simulink model "final"  (R2022a)
settings: Solver=FixedStepAuto  StartTime=0.0  StopTime=5.0  FixedStep=0.001  RelTol=1e-3
libraries: instrumentseriallib x3, slpidlib x2
settings Model: Creator=13025  LastModifiedBy=13025
settings OptimizationCC: DenormalBehavior=FlushToZero
settings DebuggingCC: ReadBeforeWriteMsg=DisableAll  WriteAfterWriteMsg=DisableAll  WriteAfterReadMsg=DisableAll

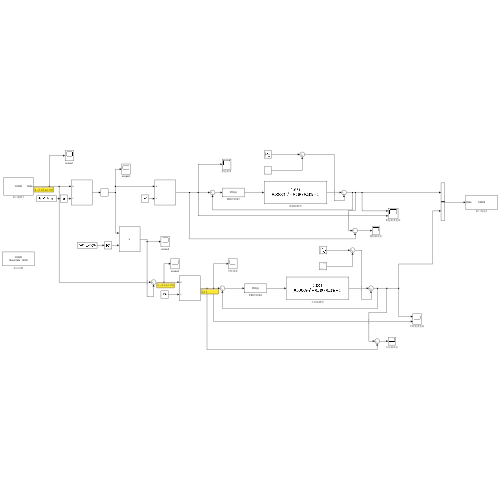
[thumbnail: Simulink's stored preview of the top-level diagram]
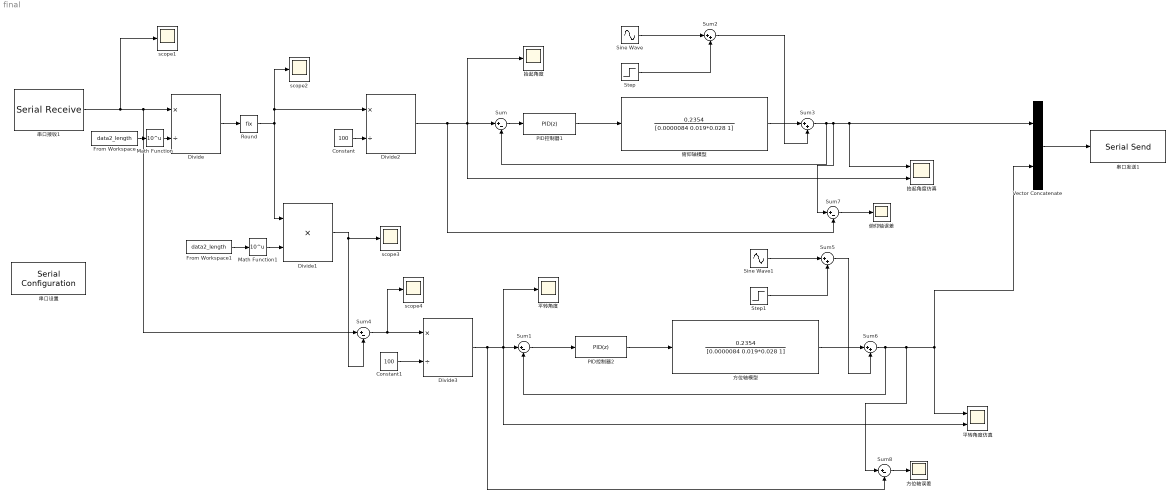
== system final ==
  Constant : Constant  Value=100
  Constant1 : Constant  Value=100
  Divide : Product  Inputs=*/  OutDataTypeStr=single  RndMeth=Round  LockScale=on
  Divide1 : Product  Inputs=**  OutDataTypeStr=single  RndMeth=Nearest  LockScale=on
  Divide2 : Product  Inputs=*/  OutDataTypeStr=double  RndMeth=Simplest
  Divide3 : Product  Inputs=*/  OutDataTypeStr=double
  From Workspace : FromWorkspace  VariableName=data2_length  OutDataTypeStr=double  SampleTime=5  OutputAfterFinalValue=Holding final value
  From Workspace1 : FromWorkspace  VariableName=data2_length  OutDataTypeStr=double  SampleTime=5  OutputAfterFinalValue=Holding final value
  Math Function : Math  Operator=10^u
  Math Function1 : Math  Operator=10^u
  PID控制器1 : slpidlib/PID Controller  Controller=PID  Form=Parallel  TimeDomain=Discrete-time  UseExternalTs=off  SampleTime=-1  IntegratorMethod=Forward Euler  FilterMethod=Forward Euler  ControllerParametersSource=internal  P=1  I=127  UseKiTs=off  D=0  N=100  UseFilter=on  TunerSelectOption=Transfer Function Based (PID Tuner App)  InitialConditionSource=internal  InitialConditionForIntegrator=0  InitialConditionForFilter=0  DifferentiatorICPrevScaledInput=0  ExternalReset=none  TrackingMode=off  Kt=1  LimitOutput=off  SatLimitsSource=internal  UpperSaturationLimit=inf  LowerSaturationLimit=-inf  LinearizeAsGain=on  AntiWindupMode=none  Kb=1  POutMin=[]  POutMax=[]  IOutMin=[]  IOutMax=[]  DOutMin=[]  DOutMax=[]  NOutMin=[]  NOutMax=[]  SumOutMin=[]  SumOutMax=[]  SaturationOutMin=[]  SaturationOutMax=[]  PParamMin=[]  PParamMax=[]  IParamMin=[]  IParamMax=[]  DParamMin=[]  DParamMax=[]  NParamMin=[]  NParamMax=[]  KbParamMin=[]  KbParamMax=[]  KtParamMin=[]  KtParamMax=[]  KbOutMin=[]  KbOutMax=[]  KtOutMin=[]  KtOutMax=[]  IntegratorOutMin=[]  IntegratorOutMax=[]  FilterOutMin=[]  FilterOutMax=[]  SumI1OutMin=[]  SumI1OutMax=[]  SumI2OutMin=[]  SumI2OutMax=[]  SumI3OutMin=[]  SumI3OutMax=[]  SumI4OutMin=[]  SumI4OutMax=[]  SumDOutMin=[]  SumDOutMax=[]  DifferentiatorOutMin=[]  DifferentiatorOutMax=[]  FilterDiffOutCoefMin=[]  FilterDiffOutCoefMax=[]  ReciprocalOutMin=[]  ReciprocalOutMax=[]  SumDenOutMin=[]  SumDenOutMax=[]  SumNumOutMin=[]  SumNumOutMax=[]  DivideOutMin=[]  DivideOutMax=[]  UdiffTsProdOutMin=[]  UdiffTsProdOutMax=[]  NTsProdOutMin=[]  NTsProdOutMax=[]  UintegralTsProdOutMin=[]  UintegralTsProdOutMax=[]  UngainTsProdOutMin=[]  UngainTsProdOutMax=[]  ClampingZeroOutDataTypeStr=Inherit: Inherit via back propagation  ClampingZeroOutMin=[]  ClampingZeroOutMax=[]  FilterDenConstantOutDataTypeStr=Inherit: Inherit via back propagation  FilterDenConstantOutMin=[]  FilterDenConstantOutMax=[]  PCopyOutDataTypeStr=Inherit: Inherit via back propagation  PCopyOutMin=[]  PCopyOutMax=[]  NCopyOutDataTypeStr=Inherit: Inherit via back propagation  NCopyOutMin=[]  NCopyOutMax=[]  IntegratorContinuousStateAttributes=''  IntegratorStateMustResolveToSignalObject=off  IntegratorRTWStateStorageClass=Auto  FilterContinuousStateAttributes=''  FilterStateMustResolveToSignalObject=off  FilterRTWStateStorageClass=Auto  ParallelPVariant=InternalParameters  IdealPVariant=Disabled  IVariant=InternalParameters  DVariant=InternalParameters  IntegratorVariant=Discrete  SatVariant=Disabled  AWVariant=Passthrough  PCopyVariant=Disabled  TRVariant=Disabled  FdbkBlocksVariant=Forward  IdealPFdbkVariant=Disabled  SatFdbkVariant=Disabled  DerivativeFilterVariant=ForwardEulerFilter  NVariant=InternalParameters  NCopyVariant=Disabled  FilterICVariant=InternalICsFilter  IntegratorICVariant=InternalICs  ExternalResetVariant=Disabled  TRSumVariant=Passthrough  SumFdbkVariant=Disabled  SumVariant=Sum_PID  TsampFilterVariant=InternalTs  TsampNgainVariant=Passthrough  TsampIntegralVariant=Passthrough  ExternalSaturationOutDataTypeStr=Inherit: Same as second input  aMode=0
  PID控制器2 : slpidlib/PID Controller  Controller=PID  Form=Parallel  TimeDomain=Discrete-time  UseExternalTs=off  SampleTime=-1  IntegratorMethod=Forward Euler  FilterMethod=Forward Euler  ControllerParametersSource=internal  P=1  I=127  UseKiTs=off  D=0  N=100  UseFilter=on  TunerSelectOption=Transfer Function Based (PID Tuner App)  InitialConditionSource=internal  InitialConditionForIntegrator=0  InitialConditionForFilter=0  DifferentiatorICPrevScaledInput=0  ExternalReset=none  TrackingMode=off  Kt=1  LimitOutput=off  SatLimitsSource=internal  UpperSaturationLimit=inf  LowerSaturationLimit=-inf  LinearizeAsGain=on  AntiWindupMode=none  Kb=1  POutMin=[]  POutMax=[]  IOutMin=[]  IOutMax=[]  DOutMin=[]  DOutMax=[]  NOutMin=[]  NOutMax=[]  SumOutMin=[]  SumOutMax=[]  SaturationOutMin=[]  SaturationOutMax=[]  PParamMin=[]  PParamMax=[]  IParamMin=[]  IParamMax=[]  DParamMin=[]  DParamMax=[]  NParamMin=[]  NParamMax=[]  KbParamMin=[]  KbParamMax=[]  KtParamMin=[]  KtParamMax=[]  KbOutMin=[]  KbOutMax=[]  KtOutMin=[]  KtOutMax=[]  IntegratorOutMin=[]  IntegratorOutMax=[]  FilterOutMin=[]  FilterOutMax=[]  SumI1OutMin=[]  SumI1OutMax=[]  SumI2OutMin=[]  SumI2OutMax=[]  SumI3OutMin=[]  SumI3OutMax=[]  SumI4OutMin=[]  SumI4OutMax=[]  SumDOutMin=[]  SumDOutMax=[]  DifferentiatorOutMin=[]  DifferentiatorOutMax=[]  FilterDiffOutCoefMin=[]  FilterDiffOutCoefMax=[]  ReciprocalOutMin=[]  ReciprocalOutMax=[]  SumDenOutMin=[]  SumDenOutMax=[]  SumNumOutMin=[]  SumNumOutMax=[]  DivideOutMin=[]  DivideOutMax=[]  UdiffTsProdOutMin=[]  UdiffTsProdOutMax=[]  NTsProdOutMin=[]  NTsProdOutMax=[]  UintegralTsProdOutMin=[]  UintegralTsProdOutMax=[]  UngainTsProdOutMin=[]  UngainTsProdOutMax=[]  ClampingZeroOutDataTypeStr=Inherit: Inherit via back propagation  ClampingZeroOutMin=[]  ClampingZeroOutMax=[]  FilterDenConstantOutDataTypeStr=Inherit: Inherit via back propagation  FilterDenConstantOutMin=[]  FilterDenConstantOutMax=[]  PCopyOutDataTypeStr=Inherit: Inherit via back propagation  PCopyOutMin=[]  PCopyOutMax=[]  NCopyOutDataTypeStr=Inherit: Inherit via back propagation  NCopyOutMin=[]  NCopyOutMax=[]  IntegratorContinuousStateAttributes=''  IntegratorStateMustResolveToSignalObject=off  IntegratorRTWStateStorageClass=Auto  FilterContinuousStateAttributes=''  FilterStateMustResolveToSignalObject=off  FilterRTWStateStorageClass=Auto  ParallelPVariant=InternalParameters  IdealPVariant=Disabled  IVariant=InternalParameters  DVariant=InternalParameters  IntegratorVariant=Discrete  SatVariant=Disabled  AWVariant=Passthrough  PCopyVariant=Disabled  TRVariant=Disabled  FdbkBlocksVariant=Forward  IdealPFdbkVariant=Disabled  SatFdbkVariant=Disabled  DerivativeFilterVariant=ForwardEulerFilter  NVariant=InternalParameters  NCopyVariant=Disabled  FilterICVariant=InternalICsFilter  IntegratorICVariant=InternalICs  ExternalResetVariant=Disabled  TRSumVariant=Passthrough  SumFdbkVariant=Disabled  SumVariant=Sum_PID  TsampFilterVariant=InternalTs  TsampNgainVariant=Passthrough  TsampIntegralVariant=Passthrough  ExternalSaturationOutDataTypeStr=Inherit: Same as second input  aMode=0
  Round : Rounding  Operator=fix
  Sine Wave : Sin  Amplitude=0.25  Frequency=2*pi*1  SampleTime=0
  Sine Wave1 : Sin  Amplitude=0.25  Frequency=2*pi*1  SampleTime=0
  Step : Step  Time=0  Before=0.25  After=0.25  SampleTime=0
  Step1 : Step  Time=0  Before=0.25  After=0.25  SampleTime=0
  Sum{,1,4,7..8} (5 alike) : Sum  Inputs=|+-
  Sum{2..3,5..6} (4 alike) : Sum  Inputs=|++
  Vector Concatenate : Concatenate
  scope{1..4} (4 alike) : Scope
  串口发送1 : instrumentseriallib/Serial Send  Priority=1  PortSel=COM2  Port=COM2  ComPort=COM2  Header=[]  Terminator=<none>  CustomTerminator=[]  EnableBlockingMode=on  SimulateUsing=Interpreted execution  BlockInModel=on  aMode=1
      settings: SourceProductBaseCode=OT,IC,MT
  串口接收1 : instrumentseriallib/Serial Receive  Priority=1  PortSel=COM2  Port=COM2  ComPort=COM2  DataType=uint32  SaveDataType=uint8  ToggleHeader=off  Header=0  ToggleTerminator=off  Terminator=<none>  CustomTerminator=[]  InputFormat=Row major  ToggleDataSize=on  DataSize=[1 1]  EnableBlockingMode=on  ActionDataUnavailable=Error  ActionWhenDataUnavailable=Error  CustomValue=0  SampleTime=0.01  SimulateUsing=Interpreted execution  BlockInModel=on  aMode=1
      settings: SourceProductBaseCode=OT,IC,MT
  串口设置 : instrumentseriallib/Serial Configuration  Priority=-200000  PortSel=COM2  Port=COM2  ComPort=COM2  BaudRate=9600  DataBits=8  Parity=none  StopBits=1  ByteOrder=little-endian  FlowControl=none  Timeout=10  SimulateUsing=Interpreted execution  BlockInModel=on  aMode=1
      settings: SourceProductBaseCode=OT,IC,MT
  俯仰轴模型 : TransferFcn  Numerator=[0.2354]  Denominator=[0.0000084 0.019*0.028 1]
  俯仰轴误差 : Scope
  平转角度 : Scope
  平转角度仿真 : Scope  NumInputPorts=2
  抬起角度 : Scope
  抬起角度仿真 : Scope  NumInputPorts=2
  方位轴模型 : TransferFcn  Numerator=[0.2354]  Denominator=[0.0000084 0.019*0.028 1]
  方位轴误差 : Scope
  wires:
  Sum/1 -> PID控制器1/1
  PID控制器1/1 -> 俯仰轴模型/1
  Sum3/1 -> Sum7/1, Vector Concatenate/1, 抬起角度仿真/1, Sum/2
  串口接收1/1 -> scope1/1, Sum4/1, Divide/1
  Divide/1 -> Round/1
  俯仰轴模型/1 -> Sum3/1
  Sine Wave/1 -> Sum2/1
  Step/1 -> Sum2/2
  Sum2/1 -> Sum3/2
  From Workspace/1 -> Math Function/1
  Math Function/1 -> Divide/2
  From Workspace1/1 -> Math Function1/1
  Math Function1/1 -> Divide1/2
  Divide1/1 -> Sum4/2, scope3/1
  Step1/1 -> Sum5/2
  方位轴模型/1 -> Sum6/1
  Sum5/1 -> Sum6/2
  Sum1/1 -> PID控制器2/1
  Sum6/1 -> Sum8/1, 平转角度仿真/1, Vector Concatenate/2, Sum1/2
  Sine Wave1/1 -> Sum5/1
  PID控制器2/1 -> 方位轴模型/1
  Divide2/1 -> Sum7/2, 抬起角度仿真/2, 抬起角度/1, Sum/1
  Constant/1 -> Divide2/2
  Constant1/1 -> Divide3/2
  Sum4/1 -> scope4/1, Divide3/1
  Divide3/1 -> Sum8/2, 平转角度仿真/2, 平转角度/1, Sum1/1
  Vector Concatenate/1 -> 串口发送1/1
  Round/1 -> scope2/1, Divide2/1, Divide1/1
  Sum7/1 -> 俯仰轴误差/1
  Sum8/1 -> 方位轴误差/1
